simulink model "MultiRateComponent"  (R2025b)
settings: Solver=FixedStepDiscrete  StartTime=0.0  StopTime=0.025  MaxStep=.0001  RelTol=1e-3  EnableMultiTasking=on
settings Model: ModifiedByFormat=The MathWorks Inc.  ExtModeAutoUpdateStatusClock=off  Creator=The MathWorks, Inc.  LastModifiedBy=The MathWorks Inc.
settings SolverCC: AlgebraicLoopSolver=TrustRegion  MaxZcPerStep=1.0
settings DataIOCC: SaveFormat=Array  SaveOutput=off  SaveTime=off  ReturnWorkspaceOutputs=off
settings OptimizationCC: DefaultParameterBehavior=Inlined  GainParamInheritBuiltInType=on  UseFloatMulNetSlope=on  UseSpecifiedMinMax=on  InlineInvariantSignals=on  PassReuseOutputArgsAs=Individual arguments  ExpressionDepthLimit=2147483647.0  ZeroExternalMemoryAtStartup=off  ZeroInternalMemoryAtStartup=off  NoFixptDivByZeroProtection=on  EfficientFloat2IntCast=on  LifeSpan=1  BufferReusableBoundary=off  OptimizeBlockOrder=speed  EfficientTunableParamExpr=on
settings DebuggingCC: SigSpecEnsureSampleTimeMsg=none  UnconnectedInputMsg=warning  UnconnectedOutputMsg=warning  UnconnectedLineMsg=warning  BusObjectLabelMismatch=none  AllowSymbolicDim=off  ModelReferenceSymbolNameMessage=none  StateNameClashWarn=warning  PregeneratedLibrarySubsystemCodeDiagnostic=none  StrictBusMsg=ErrorOnBusTreatedAsVector  SFUnexpectedBacktrackingDiag=warning  SFInvalidInputDataAccessInChartInitDiag=error  SFNoUnconditionalDefaultTransitionDiag=warning  SFExecutionAtInitializationDiag=none  ArithmeticOperatorsInVariantConditions=warning
settings HardwareCC: ProdLongLongMode=on  TargetIntDivRoundTo=Zero  TargetEndianess=LittleEndian  TargetHWDeviceType=Generic->32-bit Embedded Processor
settings ModelReferenceCC: EnableRefExpFcnMdlSchedulingChecks=on  PropagateSignalLabelsOutOfModel=off
settings SFSimCC: SimUseLocalCustomCode=off  SimParseCustomCode=off  MATLABDynamicMemAlloc=off  CustomCodeUndefinedFunction=UseInterfaceOnly
settings RTWCC: SystemTargetFile=ert.tlc  EmbeddedCoderDictionary=PlatformServices.sldd  GenCodeOnly=on  TemplateMakefile=ert_default_tmf  RTWVerbose=off  RTWUseLocalCustomCode=off  BuildConfiguration=Faster Runs  IncludeHyperlinkInReport=on  PortableWordSizes=on  DLArmComputeVersion=19.05  Description=Embedded Coder (no auto configuration)
settings CodeAppCC: ForceParamTrailComments=on  IgnoreCustomStorageClasses=off  IgnoreTestpoints=on  OperatorAnnotations=on  SimulinkDataObjDesc=on  SFDataObjDesc=on  MATLABFcnDesc=on  CustomSymbolStrGlobalVar=rt$N$M  CustomSymbolStrType=$N$M  CustomSymbolStrFcn=$N$M$F  CustomSymbolStrMacro=$N$M  InsertBlockDesc=on  StateflowObjectComments=on  MATLABSourceComments=on  EnableCustomComments=on  InternalIdentifier=Classic  ReqsInCode=on
settings ERTTargetCC: InlinedParameterPlacement=Hierarchical  ERTCustomFileTemplate=example_file_process.tlc  DynamicArrayContainerType=coder::array  TargetFcnLib=ansi_tfl_tmw.mat  UtilityFuncGeneration=Shared location  MultiwordLength=2048.0  CombineSignalStateStructs=on  SuppressErrorStatus=on  SupportNonFinite=off  SupportComplex=off
settings ConfigComp: CovMetricSettings=dw  CovSaveCumulativeToWorkspaceVar=on  CovSaveSingleToWorkspaceVar=on  CovExternalEMLEnable=off  CovSFcnEnable=off

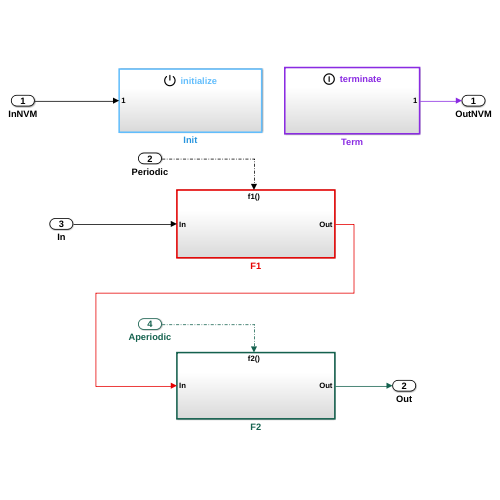
[thumbnail: Simulink's stored preview of the top-level diagram]
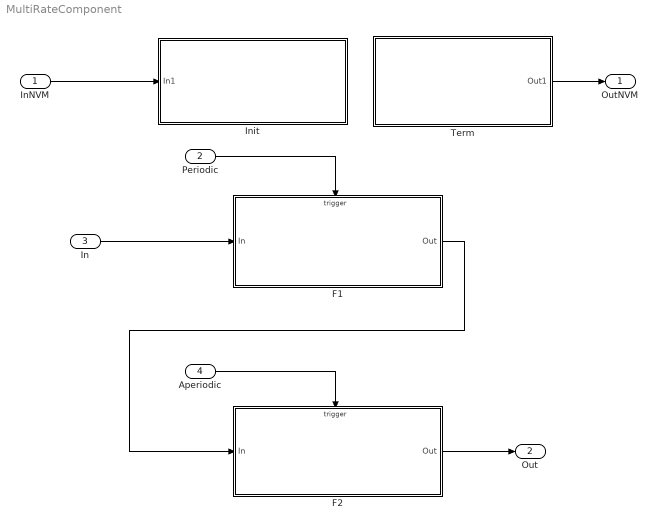
== system MultiRateComponent ==
  InNVM : Inport
  Periodic : Inport  Port=2  SampleTime=0.001  OutputFunctionCall=on
  In : Inport  Port=3
  Aperiodic : Inport  Port=4  OutputFunctionCall=on
  F1 : Subsystem  TreatAsAtomicUnit=on  RTWFcnName=foo
  F2 : Subsystem  TreatAsAtomicUnit=on  RTWFcnName=foo
  Init : Subsystem  TreatAsAtomicUnit=on  RTWFcnName=foo
  Term : Subsystem  TreatAsAtomicUnit=on  RTWFcnName=foo
  OutNVM : Outport
  Out : Outport  Port=2
  wires:
  Periodic/1 -> F1/Trigger
  InNVM/1 -> Init/1(In1)
  Term/1(Out1) -> OutNVM/1
  F2/1(Out) -> Out/1
  Aperiodic/1 -> F2/Trigger
  In/1 -> F1/1(In)
  F1/1(Out) -> F2/1(In)

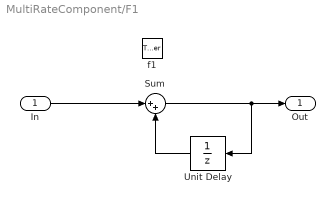
== system MultiRateComponent/F1 ==
  In : Inport
  f1 : TriggerPort  TriggerType=function-call  VariantControl=Variant  PortDimensions=1
  Sum : Sum  Inputs=|++
  Unit Delay : UnitDelay  SampleTime=-1  StateName=F1State  HasFrameUpgradeWarning=on
  Out : Outport
  wires:
  In/1 -> Sum/1
  Unit Delay/1 -> Sum/2
  Sum/1 -> Unit Delay/1, Out/1

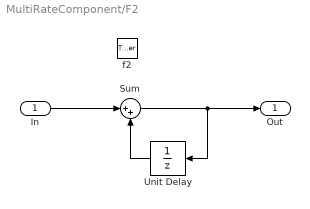
== system MultiRateComponent/F2 ==
  In : Inport
  f2 : TriggerPort  TriggerType=function-call  VariantControl=Variant  PortDimensions=1
  Sum : Sum  Inputs=|++
  Unit Delay : UnitDelay  SampleTime=-1  StateName=F2State  HasFrameUpgradeWarning=on
  Out : Outport
  wires:
  In/1 -> Sum/1
  Unit Delay/1 -> Sum/2
  Sum/1 -> Out/1, Unit Delay/1

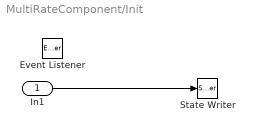
== system MultiRateComponent/Init ==
  In1 : Inport
  Event Listener : EventListener  DisableCoverage=on  EventName=reset
  State Writer : StateWriter  StateOwnerBlock=../../F1/Unit Delay  StateName=F1State
  wires:
  In1/1 -> State Writer/1

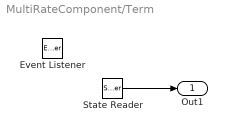
== system MultiRateComponent/Term ==
  Event Listener : EventListener  DisableCoverage=on  EventType=Terminate  EventName=reset
  State Reader : StateReader  StateOwnerBlock=../../F1/Unit Delay  StateName=F1State
  Out1 : Outport
  wires:
  State Reader/1 -> Out1/1
